simulink model "DC_motor_model_inertia_est_realtime"  (R2020b)
settings: Solver=ode3  StartTime=0.0  StopTime=20  FixedStep=0.001  RelTol=1e-3
undefined symbols (not defined in the file or in its folder): ctrl, denHwa, denHws, denHwsi, drv, National_Instruments, numHwa, numHws, numHwsi, PCI, rpm2degs, sens
libraries: sldrtlib x3, simulink x1
settings Model: ExtModeTrigDuration=30000  Creator=gioel  LastModifiedBy=saviangiul
settings DataIOCC: ReturnWorkspaceOutputs=off
settings RTWCC: Description=Simulink Desktop Real-Time  SystemTargetFile=sldrt.tlc  TemplateMakefile=sldrt.tmf  RTWCompilerOptimization=on
settings CodeAppCC: MaxIdLength=95
settings SimulinkDesktopRealTimeCC: TargetPreCompLibLocation=C:\Program Files\MATLAB\R2020b\toolbox\sldrt\lib\win64

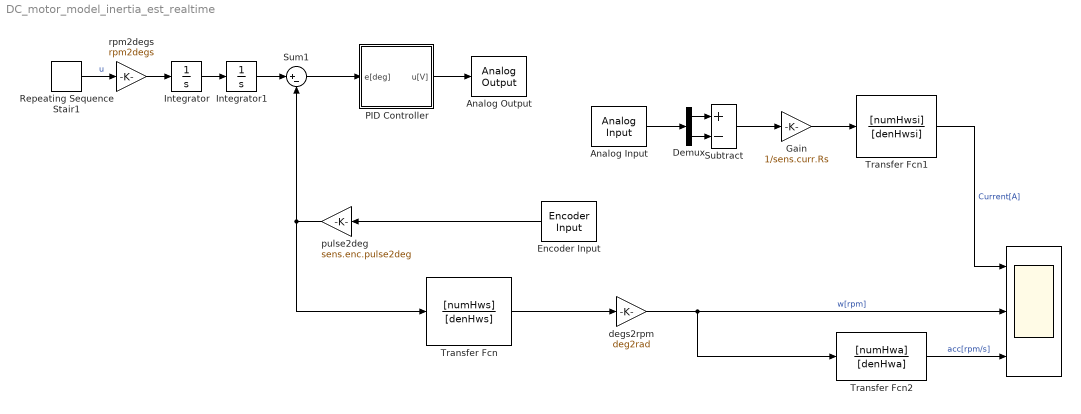
== system DC_motor_model_inertia_est_realtime ==
  " " : Scope  NumInputPorts=3
  Analog Input : sldrtlib/Analog Input  SampleTime=0.001  MaxMissedTicks=10  ShowMissedTicks=off  YieldWhenWaiting=off  DrvName=National_Instruments/PCI-6221  DrvAddress=4294967295  DrvOptions=[0 0 0 2 0]  Channels=[1 2]  RangeMode=1  VoltRange=1  DataType=1
      settings: AttributesFormatString=National Instruments\nPCI-6221 [auto]
  Analog Output : sldrtlib/Analog Output  SampleTime=0.001  MaxMissedTicks=10  ShowMissedTicks=off  YieldWhenWaiting=off  DrvName=National_Instruments/PCI-6221  DrvAddress=4294967295  DrvOptions=[0 0 0 2 0]  Channels=1  RangeMode=1  VoltRange=1  InitialValue=0  FinalValue=0
      settings: AttributesFormatString=National Instruments\nPCI-6221 [auto]
  Demux : Demux  Outputs=2
  Encoder Input : sldrtlib/Encoder Input  SampleTime=0.001  MaxMissedTicks=10  ShowMissedTicks=off  YieldWhenWaiting=off  DrvName=National_Instruments/PCI-6221  DrvAddress=4294967295  DrvOptions=[0 0 0 2 0]  Channels=1  QuadMode=3  IndexPulse=1  InputFilter=Inf  DataType=1
      settings: AttributesFormatString=National Instruments\nPCI-6221 [auto]
  Gain : Gain  Gain=1/sens.curr.Rs
  Integrator : Integrator
  Integrator1 : Integrator
  PID Controller : Subsystem
  Repeating Sequence Stair1 : simulink/Sources/Repeating Sequence Stair  OutValues=[450 -450].'  tsamp=1  OutMin=[]  OutMax=[]  OutDataTypeStr=double  OutputDataTypeScalingMode=double  OutDataType=fixdt(0,8)  ConRadixGroup=Best Precision: Vector-wise  OutScaling=2^-12
  Subtract : Sum  Inputs=+-
  Sum1 : Sum  Inputs=|+-
  Transfer Fcn : TransferFcn  Numerator=[numHws]  Denominator=[denHws]
  Transfer Fcn1 : TransferFcn  Numerator=[numHwsi]  Denominator=[denHwsi]
  Transfer Fcn2 : TransferFcn  Numerator=[numHwa]  Denominator=[denHwa]
  degs2rpm : Gain  Gain=deg2rad
  pulse2deg : Gain  Gain=sens.enc.pulse2deg
  rpm2degs : Gain  Gain=rpm2degs
  wires:
  Sum1/1 -> PID Controller/1(e[deg])
  PID Controller/1(u[V]) -> Analog Output/1
  Encoder Input/1 -> pulse2deg/1
  pulse2deg/1 -> Transfer Fcn/1, Sum1/2
  degs2rpm/1 -> " "/2, Transfer Fcn2/1  "w[rpm]"
  Transfer Fcn/1 -> degs2rpm/1
  Integrator/1 -> Integrator1/1
  Transfer Fcn1/1 -> " "/1  "Current[A]"
  Gain/1 -> Transfer Fcn1/1
  Analog Input/1 -> Demux/1
  Demux/1 -> Subtract/1
  Subtract/1 -> Gain/1
  Demux/2 -> Subtract/2
  Transfer Fcn2/1 -> " "/3  "acc[rpm/s]"
  Repeating Sequence Stair1/1 -> rpm2degs/1  "u"
  rpm2degs/1 -> Integrator/1
  Integrator1/1 -> Sum1/1

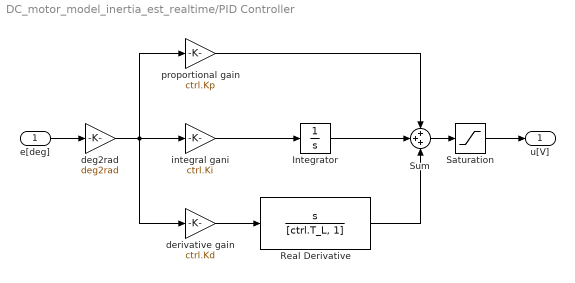
== system DC_motor_model_inertia_est_realtime/PID Controller ==
  e[deg] : Inport
  Integrator : Integrator
  Real Derivative : TransferFcn  Numerator=[1 0]  Denominator=[ctrl.T_L, 1]
  Saturation : Saturate  UpperLimit=drv.outmax  LowerLimit=-drv.outmax
  Sum : Sum  Inputs=+++
  deg2rad : Gain  Gain=deg2rad
  derivative gain : Gain  Gain=ctrl.Kd
  integral gani : Gain  Gain=ctrl.Ki
  proportional gain : Gain  Gain=ctrl.Kp
  u[V] : Outport
  wires:
  Sum/1 -> Saturation/1
  Saturation/1 -> u[V]/1
  derivative gain/1 -> Real Derivative/1
  Real Derivative/1 -> Sum/3
  Integrator/1 -> Sum/2
  integral gani/1 -> Integrator/1
  proportional gain/1 -> Sum/1
  e[deg]/1 -> deg2rad/1
  deg2rad/1 -> derivative gain/1, proportional gain/1, integral gani/1
